simulink model "Longitudinal_Autopilot"  (R2019a)
settings: Solver=VariableStepAuto  StartTime=0.0  StopTime=tfinal  RelTol=1e-3
undefined symbols (not defined in the file or in its folder): A_Long_Full, B_Long_Full, C_Long_Full, D_Long_Full, h_command, K_d_theta, theta0, u0, u_command, w0, z0
libraries: cstblocks x5, simulink x1, SignalEditorBlockLib x1
settings Model: Creator=pc  LastModifiedBy=Ahmed Essam
settings DataIOCC: SaveFormat=Array
settings DebuggingCC: ArithmeticOperatorsInVariantConditions=warning
settings SFSimCC: SimUseLocalCustomCode=off
settings RTWCC: RTWUseLocalCustomCode=off
settings CodeAppCC: StateflowObjectComments=on

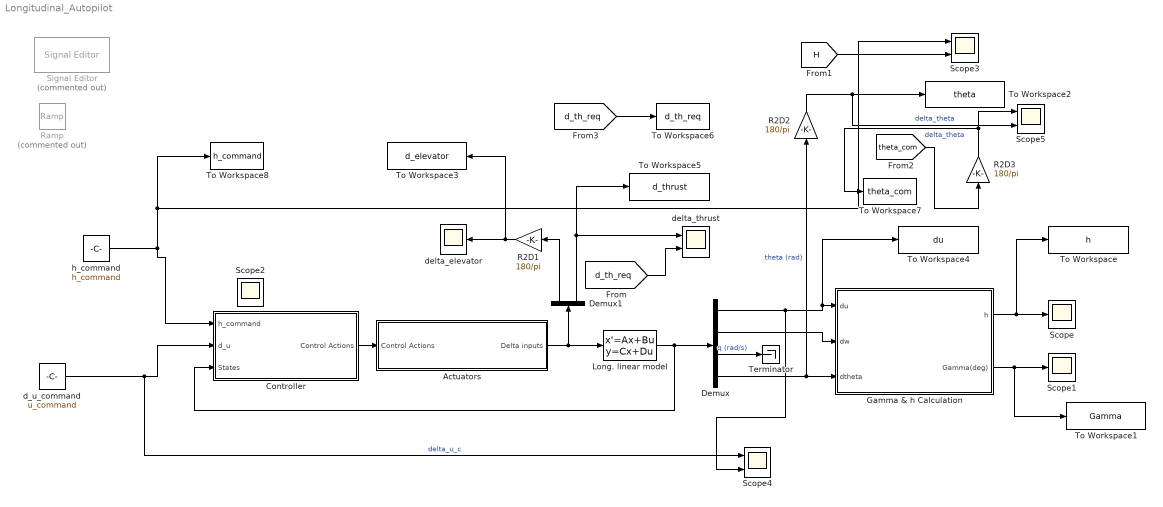
== system Longitudinal_Autopilot ==
  Actuators : Subsystem
  Controller : Subsystem
  Demux : Demux
  Demux1 : Demux  Outputs=2
  Gamma & h Calculation : Subsystem
  Long. linear model : StateSpace  A=A_Long_Full  B=B_Long_Full  C=C_Long_Full  D=D_Long_Full  InitialCondition=0
  R2D1 : Gain  Gain=180/pi
  R2D2 : Gain  Gain=180/pi
  R2D3 : Gain  Gain=180/pi
  Ramp : simulink/Sources/Ramp  Commented=on  slope=20  start=0  InitialOutput=0
  Scope : Scope
  Scope1 : Scope
  Scope3 : Scope  NumInputPorts=2
  Scope4 : Scope  NumInputPorts=2
  Scope5 : Scope  NumInputPorts=2
  Signal Editor : SignalEditorBlockLib/Signal Editor  Commented=on  FileName=input.mat  ActiveScenario=Scenario  ActiveSignal=Signal 1  IsBus=off  OutputBusObjectStr=Bus: BusObject  SampleTime=0  Interpolate=off  ZeroCross=off  OutputAfterFinalValue=Setting to zero  Unit=inherit  PreserveSignalName=on
      settings: SourceProductName=Simulink
  Terminator : Terminator
  To Workspace : ToWorkspace  VariableName=h  SampleTime=-1
  To Workspace1 : ToWorkspace  VariableName=Gamma  SampleTime=-1
  To Workspace2 : ToWorkspace  VariableName=theta  SampleTime=-1
  To Workspace3 : ToWorkspace  VariableName=d_elevator  SampleTime=-1
  To Workspace4 : ToWorkspace  VariableName=du  SampleTime=-1
  To Workspace5 : ToWorkspace  VariableName=d_thrust  SampleTime=-1
  To Workspace6 : ToWorkspace  VariableName=d_th_req  SampleTime=-1
  To Workspace7 : ToWorkspace  VariableName=theta_com  SampleTime=-1
  To Workspace8 : ToWorkspace  VariableName=h_command  SampleTime=-1
  d_u_command : Constant  Value=u_command
  delta_elevator : Scope
  delta_thrust : Scope  NumInputPorts=2
  h_command : Constant  Value=h_command
  Scope2 : Scope
  wires:
  Demux/4 -> Gamma & h Calculation/3(dtheta), R2D2/1  "theta (rad)"
  Long. linear model/1 -> Controller/3(States), Demux/1
  Demux/1 -> Scope4/2, To Workspace4/1, Gamma & h Calculation/1(du)
  Demux/2 -> Gamma & h Calculation/2(dw)
  Gamma & h Calculation/1(h) -> To Workspace/1, Scope/1
  Gamma & h Calculation/2(Gamma(deg)) -> Scope1/1, To Workspace1/1
  R2D1/1 -> To Workspace3/1, delta_elevator/1
  R2D2/1 -> Scope5/2, To Workspace2/1  "delta_theta"
  Controller/1(Control Actions) -> Actuators/1(Control Actions)
  Demux/3 -> Terminator/1  "q (rad/s)"
  Actuators/1("Delta inputs ") -> Long. linear model/1, Demux1/1
  Demux1/1 -> R2D1/1
  d_u_command/1 -> Scope4/1, Controller/2(d_u)  "delta_u_c"
  Demux1/2 -> delta_thrust/1, To Workspace5/1
  [d_th_req] -> delta_thrust/2
  [H] -> Scope3/2
  [theta_com] -> R2D3/1
  R2D3/1 -> To Workspace7/1, Scope5/1  "delta_theta"
  [d_th_req] -> To Workspace6/1
  h_command/1 -> Controller/1(h_command), To Workspace8/1, Scope3/1

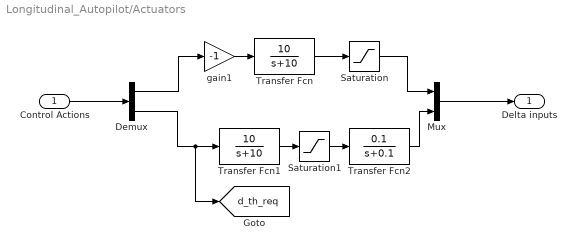
== system Longitudinal_Autopilot/Actuators ==
  Control Actions : Inport
  Demux : Demux  Outputs=2
  Mux : Mux  Inputs=2
  Saturation : Saturate  UpperLimit=25*pi/180  LowerLimit=-25*pi/180
  Saturation1 : Saturate  UpperLimit=3700  LowerLimit=-2*3700
  Transfer Fcn : TransferFcn  Numerator=[10]  Denominator=[1 10]
  Transfer Fcn1 : TransferFcn  Numerator=[10]  Denominator=[1 10]
  Transfer Fcn2 : TransferFcn  Numerator=[0.1]  Denominator=[1 0.1]
  gain1 : Gain  Gain=-1
  "Delta inputs " : Outport  VectorParamsAs1DForOutWhenUnconnected=on
  tag scope: d_th_req=global
  wires:
  Saturation/1 -> Mux/1
  Transfer Fcn/1 -> Saturation/1
  gain1/1 -> Transfer Fcn/1
  Control Actions/1 -> Demux/1
  Demux/1 -> gain1/1
  Demux/2 -> [d_th_req], Transfer Fcn1/1
  Transfer Fcn2/1 -> Mux/2
  Mux/1 -> "Delta inputs "/1
  Transfer Fcn1/1 -> Saturation1/1
  Saturation1/1 -> Transfer Fcn2/1

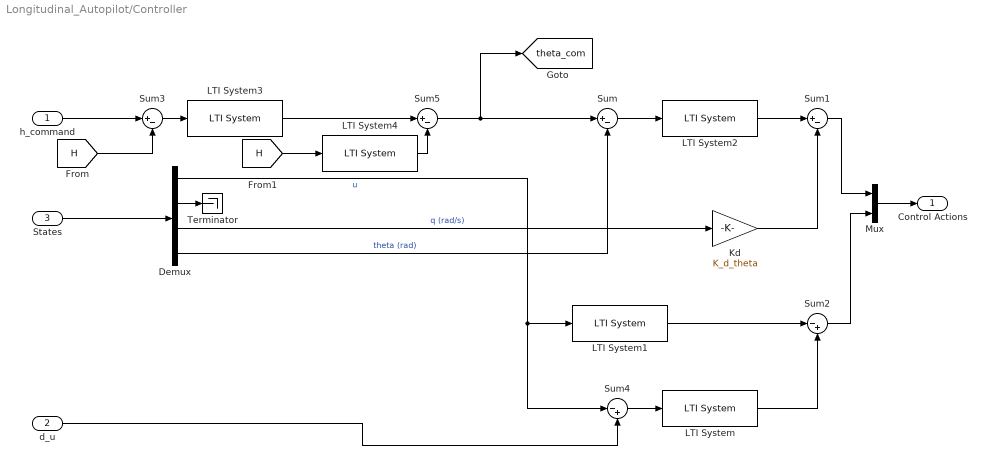
== system Longitudinal_Autopilot/Controller ==
  h_command : Inport
  d_u : Inport  Port=2
  States : Inport  Port=3
  Demux : Demux
  Kd : Gain  Gain=K_d_theta
  LTI System : cstblocks/LTI System  sys=PI_vel  IC=[]
  LTI System1 : cstblocks/LTI System  sys=Compensator_vel  IC=[]
  LTI System2 : cstblocks/LTI System  sys=PI_Pitch  IC=[]
  LTI System3 : cstblocks/LTI System  sys=PI_Alt  IC=[]
  LTI System4 : cstblocks/LTI System  sys=P_Alt  IC=[]
  Mux : Mux  Inputs=2
  Sum{,1,3,5} (4 alike) : Sum  Inputs=|+-
  Sum2 : Sum  Inputs=|-+
  Sum4 : Sum  Inputs=|-+
  Terminator : Terminator
  Control Actions : Outport  VectorParamsAs1DForOutWhenUnconnected=on
  tag scope: theta_com=global
  wires:
  Kd/1 -> Sum1/2
  LTI System2/1 -> Sum1/1
  Sum/1 -> LTI System2/1
  Sum1/1 -> Mux/1
  Demux/4 -> Sum/2  "theta (rad)"
  States/1 -> Demux/1
  Demux/3 -> Kd/1  "q (rad/s)"
  Demux/1 -> Sum4/1, LTI System1/1  "u"
  Mux/1 -> Control Actions/1
  Sum4/1 -> LTI System/1
  Demux/2 -> Terminator/1
  d_u/1 -> Sum4/2
  LTI System1/1 -> Sum2/1
  LTI System/1 -> Sum2/2
  Sum2/1 -> Mux/2
  [H] -> Sum3/2
  h_command/1 -> Sum3/1
  Sum3/1 -> LTI System3/1
  LTI System3/1 -> Sum5/1
  Sum5/1 -> [theta_com], Sum/1
  [H] -> LTI System4/1
  LTI System4/1 -> Sum5/2

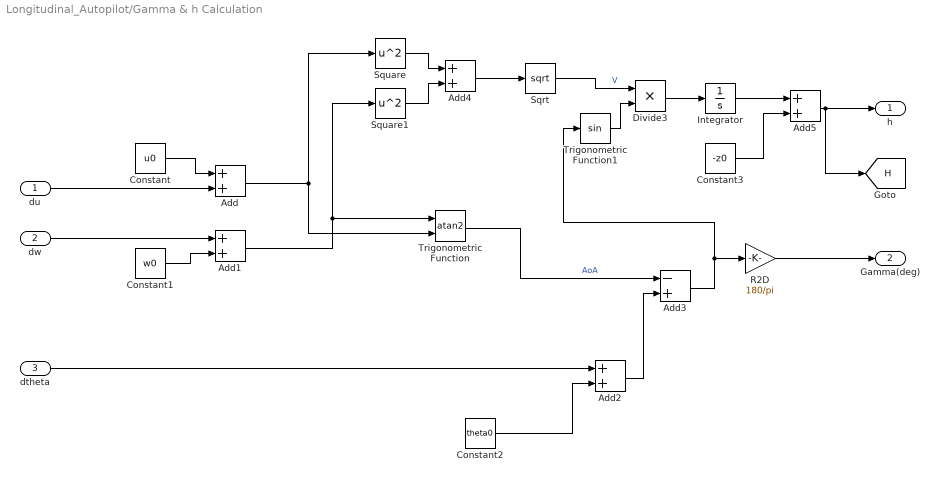
== system Longitudinal_Autopilot/Gamma & h Calculation ==
  du : Inport
  dw : Inport  Port=2
  dtheta : Inport  Port=3
  Add{,1..2,4..5} (5 alike) : Sum
  Add3 : Sum  Inputs=-+
  Constant : Constant  Value=u0
  Constant1 : Constant  Value=w0
  Constant2 : Constant  Value=theta0
  Constant3 : Constant  Value=-z0
  Divide3 : Product  Inputs=**
  Integrator : Integrator
  R2D : Gain  Gain=180/pi
  Sqrt : Sqrt  SaturateOnIntegerOverflow=on
  Square : Math  Operator=square  SaturateOnIntegerOverflow=on
  Square1 : Math  Operator=square  SaturateOnIntegerOverflow=on
  Trigonometric Function : Trigonometry  Operator=atan2
  Trigonometric Function1 : Trigonometry
  h : Outport  VectorParamsAs1DForOutWhenUnconnected=on
  Gamma(deg) : Outport  Port=2  VectorParamsAs1DForOutWhenUnconnected=on
  tag scope: H=global
  wires:
  Add1/1 -> Trigonometric Function/1, Square1/1
  dw/1 -> Add1/1
  Trigonometric Function/1 -> Add3/1  "AoA"
  Add3/1 -> Trigonometric Function1/1, R2D/1
  Constant3/1 -> Add5/2
  Divide3/1 -> Integrator/1
  Sqrt/1 -> Divide3/1  "V"
  Constant/1 -> Add/1
  Trigonometric Function1/1 -> Divide3/2
  Integrator/1 -> Add5/1
  Add2/1 -> Add3/2
  Square/1 -> Add4/1
  du/1 -> Add/2
  Square1/1 -> Add4/2
  Constant1/1 -> Add1/2
  Constant2/1 -> Add2/2
  Add/1 -> Trigonometric Function/2, Square/1
  Add4/1 -> Sqrt/1
  R2D/1 -> Gamma(deg)/1
  dtheta/1 -> Add2/1
  Add5/1 -> [H], h/1
